simulink model "Model_with_Load"  (R2018b)
settings: Solver=VariableStepAuto  StartTime=0.0  StopTime=0.2  RelTol=1e-3
undefined symbols (not defined in the file): Ion, Lithium
libraries: powerlib x22, powerlib_meascontrol x3, electricdrivelib x1
settings Model: Creator=DELL  LastModifiedBy=DELL
settings DebuggingCC: UnconnectedInputMsg=none  UnconnectedOutputMsg=none  UnconnectedLineMsg=none

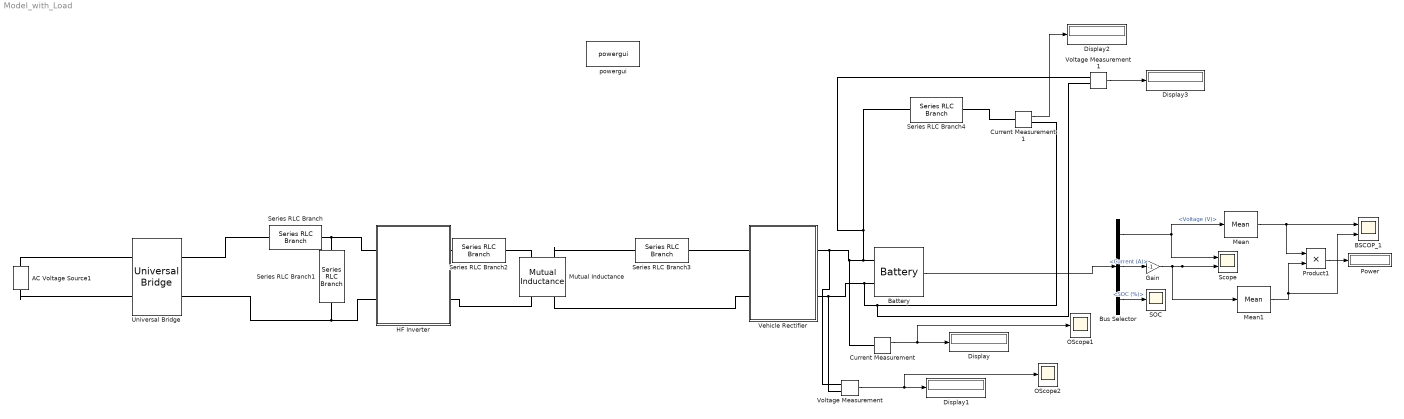
== system Model_with_Load ==
  AC Voltage Source1 : powerlib/Electrical Sources/AC Voltage Source  Amplitude=312  Phase=0  Frequency=50  SampleTime=0  Measurements=Voltage  BusType=swing  Pref=10e3  Qref=0  Qmin=-inf  Qmax=+inf
  BSCOP_1 : Scope  NumInputPorts=2
  Battery : electricdrivelib/Extra Sources/Battery  BatType=Lithium-Ion  ShowTempParam=off  ThermalPreset=no  ShowAgeParam=off  NomV=360  NomQ=100  SOC=80  Batt_Tr=10  PresetModel=on  MaxQ=100  MinV=270  FullV=419.0354  Dis_rate=43.4783  R=0.036  Normal_OP=90.4348  expZone="[388.9389      4.913043]"  current=[6.5 13 32.5]  Units=Time  Tci=20  NomT=20  T2=-30  MaxQ2=4.8  FullV2=7.1  Normal_OP2=5.655  expZone2="[6.58           1]"  Rca=0.6  ti=2000  Dp=0  Neq0=0  Tsim=1e6  Ta1=25  Qeol=5.4*0.9  Reol=0.013333*1.2  Char_age=[2.3478, 3]  Dis_age=[2.3478, 10]  N1=1500  N2=10500  N3=1000  N4=1400  Ta2=45  N5=950
  Bus Selector : BusSelector  OutputSignals=Voltage (V),Current (A),SOC (%)
  Current Measurement : powerlib/Measurements/Current Measurement  PhasorSimulation=off  OutputType=Magnitude  PSBequivalent=0
  Current Measurement1 : powerlib/Measurements/Current Measurement  PhasorSimulation=off  OutputType=Magnitude  PSBequivalent=0
  Display{,1..3} (4 alike) : Display
  Gain : Gain  Gain=-1
  HF Inverter : Subsystem
  Mean : powerlib_meascontrol/Measurements/Mean  Freq=50  Vinit=0  Ts=0
  Mean1 : powerlib_meascontrol/Measurements/Mean  Freq=50  Vinit=0  Ts=0
  Mutual Inductance : powerlib/Elements/Mutual Inductance  LConnTagsString=a|b  RConnTagsString=A|B  TypeOfMutual=Two or three windings with equal mutual terms  NumberOfWindings=3  SelfImpedance1=[1e-3 266.16e-6]  SelfImpedance2=[1e-3 256.79e-6]  ThreeWindings=off  SelfImpedance3=[ 1.1 1.1e-03]  MutualImpedance=[0 85.46e-6]  InductanceMatrix="[1.0 0.9  0.9 ;  0.9 1.0  0.9;  0.9 0.9 1.0 ] * 1e-3"  ResistanceMatrix="[1.0 0.9  0.9 ;  0.9 1.0  0.9;  0.9 0.9 1.0 ]"  Measurements=None
      settings: AttributesFormatString=\n  SourceProductName=Simscape Power Systems  SourceProductBaseCode=PS
  OScope1 : Scope
  OScope2 : Scope
  Power : Display
  Product1 : Product
  SOC : Scope
  Scope : Scope  NumInputPorts=2
  Series RLC Branch : powerlib/Elements/Series RLC Branch  LConnTagsString=__new0  RConnTagsString=__new0  BranchType=L  Resistance=1  Inductance=10e-3  SetiL0=off  InitialCurrent=0  Capacitance=1e-6  Setx0=off  InitialVoltage=0  Measurements=Branch current
  Series RLC Branch1 : powerlib/Elements/Series RLC Branch  LConnTagsString=__new0  RConnTagsString=__new0  BranchType=C  Resistance=1  Inductance=10e-3  SetiL0=off  InitialCurrent=0  Capacitance=300e-6  Setx0=off  InitialVoltage=0  Measurements=None
  Series RLC Branch2 : powerlib/Elements/Series RLC Branch  LConnTagsString=__new0  RConnTagsString=__new0  BranchType=C  Resistance=1  Inductance=10e-3  SetiL0=off  InitialCurrent=0  Capacitance=105.74e-9  Setx0=off  InitialVoltage=0  Measurements=Branch current
  Series RLC Branch3 : powerlib/Elements/Series RLC Branch  LConnTagsString=__new0  RConnTagsString=__new0  BranchType=C  Resistance=1  Inductance=10e-3  SetiL0=off  InitialCurrent=0  Capacitance=109.69e-9  Setx0=off  InitialVoltage=0  Measurements=Branch current
  Series RLC Branch4 : powerlib/Elements/Series RLC Branch  LConnTagsString=__new0  RConnTagsString=__new0  BranchType=R  Resistance=0.4  Inductance=10e-3  SetiL0=off  InitialCurrent=0  Capacitance=109.69e-9  Setx0=off  InitialVoltage=0  Measurements=Branch voltage and current
  Universal Bridge : powerlib/Power Electronics/Universal Bridge  Arms=2  SnubberResistance=1e5  SnubberCapacitance=inf  Device=Diodes  Ron=1e-3  Lon=0  ForwardVoltages="[  0  0  ]"  ForwardVoltage=0  GTOparameters=[ 10e-6 , 20e-6 ]  IGBTparameters=[ 1e-6 , 2e-6 ]  Measurements=All voltages and currents  Measurements_2=None  converterType=Rectifier
  Vehicle Rectifier : Subsystem
  Voltage Measurement : powerlib/Measurements/Voltage Measurement  PhasorSimulation=off  OutputType=Magnitude  PSBequivalent=0
  Voltage Measurement1 : powerlib/Measurements/Voltage Measurement  PhasorSimulation=off  OutputType=Magnitude  PSBequivalent=0
  powergui : powerlib/powergui  Priority=1  SimulationMode=Continuous  SampleTime=50e-6  frequency=60  Iterations=50  frequencyindice=50  Pbase=100e6  ErrMax=1e-4  UnitsV=kV  UnitsW=MW  buscounter=0  FunctionMessages=off  echomessages=off  EnableUseOfTLC=off  CurrentSourceSwitches=off  DisableSnubberDevices=off  DisableRonSwitches=off  DisableVfSwitches=off  DisplayEquations=off  SolverType=Tustin/Backward Euler (TBE)  Interpol=off  ExternalGateDelay=off  methode=off  Ts=100  x0status=blocks  SPID=on  SwTol=0  HookPort=off  RestoreLinks=warning  ResistiveCurrentMeasurement=off  Frange=[0:2:500]  Ylog=off  Xlog=on  ShowGrid=off  save=off  variable=ZData  structure=0  ZoomFFT=off  StartTime=0.0  cycles=1  DisplayStyle=1  fundamental=60  FreqAxis=off  MaxFrequency=1000  frequencyindicesteady=1  RmsSteady=1  display=off
  wires:
  Gain/1 -> Mean1/1, Scope/2
  Bus Selector/1 -> Scope/1, Mean/1  "<Voltage (V)>"
  Bus Selector/3 -> SOC/1  "<SOC (%)>"
  Bus Selector/2 -> Gain/1  "<Current (A)>"
  Product1/1 -> Power/1
  Mean1/1 -> Product1/2, BSCOP_1/2
  Mean/1 -> Product1/1, BSCOP_1/1
  Voltage Measurement/1 -> OScope2/1, Display1/1
  Battery/1 -> Bus Selector/1
  Current Measurement/1 -> OScope1/1, Display/1
  Current Measurement1/1 -> Display2/1
  Voltage Measurement1/1 -> Display3/1
  connections:
  AC Voltage Source1/LConn1 -- Universal Bridge/LConn2
  Universal Bridge/RConn2 -- Series RLC Branch1/RConn1 -- HF Inverter/LConn2
  Series RLC Branch/RConn1 -- Series RLC Branch1/LConn1 -- HF Inverter/LConn1
  Series RLC Branch2/LConn1 -- HF Inverter/RConn1
  Series RLC Branch2/RConn1 -- Mutual Inductance/LConn1
  Mutual Inductance/RConn1 -- HF Inverter/RConn2
  Vehicle Rectifier/LConn1 -- Series RLC Branch3/RConn1
  Mutual Inductance/RConn2 -- Vehicle Rectifier/LConn2
  Mutual Inductance/LConn2 -- Series RLC Branch3/LConn1
  Vehicle Rectifier/RConn1 -- Voltage Measurement/LConn1 -- Current Measurement/LConn1 -- Series RLC Branch4/LConn1 -- Voltage Measurement1/LConn1 -- Battery/LConn1
  Vehicle Rectifier/RConn2 -- Voltage Measurement/LConn2 -- Current Measurement1/RConn1 -- Voltage Measurement1/LConn2 -- Battery/LConn2
  AC Voltage Source1/RConn1 -- Universal Bridge/LConn1
  Universal Bridge/RConn1 -- Series RLC Branch/LConn1
  Current Measurement1/LConn1 -- Series RLC Branch4/RConn1

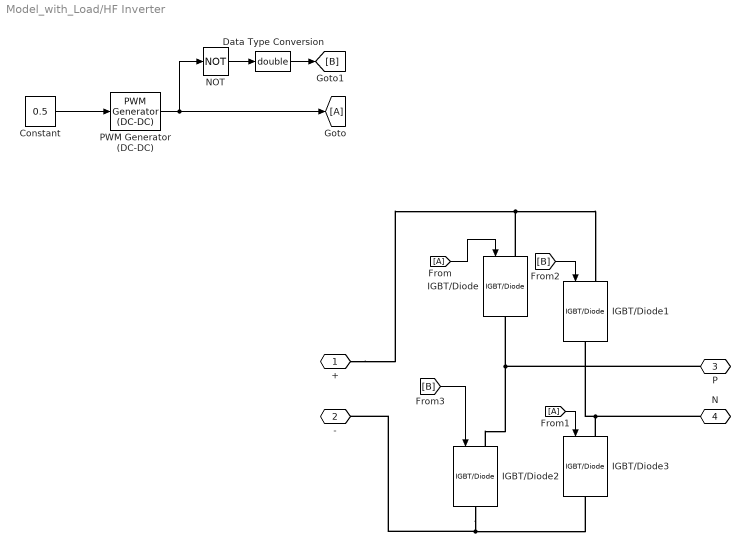
== system Model_with_Load/HF Inverter ==
  Constant : Constant  Value=0.5
  Data Type Conversion : DataTypeConversion  OutDataTypeStr=double
  IGBT/Diode{,1..3} (4 alike) : powerlib/Power Electronics/IGBT//Diode  Ron=1e-3  Rs=1e5  Cs=inf  Measurements=off
  "NOT " : Logic  Operator=NOT  IconShape=distinctive  AllPortsSameDT=off  OutDataTypeStr=boolean
  PWM Generator (DC-DC) : powerlib_meascontrol/Pulse & Signal Generators/PWM Generator (DC-DC)  Fsw=30000  Ts=0
  + : PMIOPort  Side=Left
  - : PMIOPort  Port=2  Side=Left
  P : PMIOPort  Port=3  Side=Right
  N : PMIOPort  Port=4  Side=Right
  wires:
  [B] -> IGBT/Diode1/1
  [B] -> IGBT/Diode2/1
  [A] -> IGBT/Diode3/1
  [A] -> IGBT/Diode/1
  "NOT "/1 -> Data Type Conversion/1
  Constant/1 -> PWM Generator (DC-DC)/1
  Data Type Conversion/1 -> [B]
  PWM Generator (DC-DC)/1 -> "NOT "/1, [A]
  connections:
  IGBT/Diode/LConn1 -- +/RConn1 -- IGBT/Diode1/LConn1
  IGBT/Diode3/LConn1 -- N/RConn1 -- IGBT/Diode1/RConn1
  IGBT/Diode2/RConn1 -- -/RConn1 -- IGBT/Diode3/RConn1
  IGBT/Diode2/LConn1 -- P/RConn1 -- IGBT/Diode/RConn1

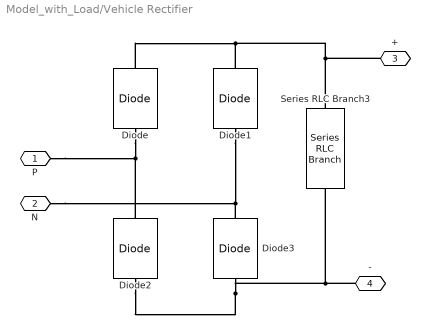
== system Model_with_Load/Vehicle Rectifier ==
  Diode{,1..3} (4 alike) : powerlib/Power Electronics/Diode  Ron=0.001  Lon=0  Vf=0.8  IC=0  UseSnubber=0  Rs=500  Cs=250e-9  Measurements=off
  Series RLC Branch3 : powerlib/Elements/Series RLC Branch  LConnTagsString=__new0  RConnTagsString=__new0  BranchType=C  Resistance=1  Inductance=10e-3  SetiL0=off  InitialCurrent=0  Capacitance=300e-6  Setx0=off  InitialVoltage=0  Measurements=Branch voltage
  P : PMIOPort  Side=Left
  N : PMIOPort  Port=2  Side=Left
  + : PMIOPort  Port=3  Side=Right
  - : PMIOPort  Port=4  Side=Right
  connections:
  Diode1/RConn1 -- Diode/RConn1 -- +/RConn1 -- Series RLC Branch3/LConn1
  Diode/LConn1 -- P/RConn1 -- Diode2/RConn1
  Diode3/LConn1 -- Diode2/LConn1 -- -/RConn1 -- Series RLC Branch3/RConn1
  N/RConn1 -- Diode3/RConn1 -- Diode1/LConn1
